simulink model "W01_Base_Map_cs"  (R2019a)
settings: Solver=FixedStepDiscrete  StartTime=0.0  StopTime=40  FixedStep=1/20  RelTol=1e-3
PreLoadFcn:
  | mbxruntime.callbacks.PreLoadFcn(bdroot);
  | check_NUTS_defined
  | model_closed = 0;
  | assignin('base',['model_closed_' bdroot],false);
PostLoadFcn:
  | mbxruntime.callbacks.PostLoadFcn(bdroot);
InitFcn:
  | mbxruntime.callbacks.InitFcn(bdroot);
StartFcn:
  | mbxruntime.callbacks.StartFcn(bdroot);
StopFcn:
  | mbxruntime.callbacks.StopFcn(bdroot);;
  | 
model workspace: external: MAT-File .\W01_Base_Map_cs_hws.mat (data not in the file)
undefined symbols (not defined in the file or in its folder): DiscIntNeverNeededParam, InitImageOutputDir, mbxruntime, tabledata, W01_Base_Map_cs_328ec7e3a8cd5b54, W01_Base_Map_cs_423c72fa17799c7f, W01_Base_Map_cs_514c2dea2cdbe680, W01_Base_Map_cs_51d6e6e467bedba1, W01_Base_Map_cs_563ebd29d1fd6c09, W01_Base_Map_cs_57ea59d0358dab77, W01_Base_Map_cs_669d1acb174df2b9, W01_Base_Map_cs_774a522413284ef7, W01_Base_Map_cs_9538d35a279fbe4e, W01_Base_Map_cs_9f504bb84aebc2fd, W01_Base_Map_cs_a242ed7539861165, W01_Base_Map_cs_ae41b72d7e14f81d, W01_Base_Map_cs_Audi_A8_Sedan_1_Path_pathUniqueID, W01_Base_Map_cs_b5931a786e299506, W01_Base_Map_cs_b7f45a070fa6e639, W01_Base_Map_cs_c02beb48492dde12, W01_Base_Map_cs_c75b75e9f6b035bf, W01_Base_Map_cs_cf83ac8e8b053cbf, W01_Base_Map_cs_Child_RegularAni_1_Path_pathUniqueID, W01_Base_Map_cs_Child_RegularAni_2_Path_pathUniqueID, W01_Base_Map_cs_Citroen_C3_Hatchback_1_Path_pathUniqueID, W01_Base_Map_cs_d4423fcf1c0d6fc4, W01_Base_Map_cs_df133aa86d9852fe, W01_Base_Map_cs_Female_RegularAni_1_Path_pathUniqueID, W01_Base_Map_cs_Male_RegularAni_1_Path_pathUniqueID, W01_Base_Map_cs_Male_RegularAni_2_Path_pathUniqueID
libraries: simulink_extras x41, adeye_lib x15, simulink x10, dspindex x6, PreScanSimulinkLibrary x4, sharedtransform x3, robotcorelib x1, PreScanUsefulBlocks x1
(part 9 of 11)

== system W01_Base_Map_cs/Ford_Fiesta_Hatchback_1/AIR_1_Demux ==
  AIR : Inport
  Activate_Switch : Subsystem
      mask Display: text(5,10,'')
  Bus Selector : BusSelector  OutputSignals=DATA.Range,DATA.Azimuth,DATA.Elevation,DATA.ID,DATA.Velocity,DATA.Heading
  Data Type Conversion : DataTypeConversion  OutDataTypeStr=double
  For Iterator : ForIterator  ResetStates=reset  IterationLimit=detectableObjects
  Selector : Selector  InputPortWidth=detectableObjects  IndexOptions=Index vector (port)  Indices=[1 3]  OutputSizes=1
  Signal2ArrayOfSignals1 : Subsystem  mask{VECTORLENGTH=detectableObjects}
      mask prompts: VECTORLENGTH "Length of vector"
  Signal2ArrayOfSignals2 : Subsystem  mask{VECTORLENGTH=detectableObjects}
      mask prompts: VECTORLENGTH "Length of vector"
  Signal2ArrayOfSignals3 : Subsystem  mask{VECTORLENGTH=detectableObjects}
      mask prompts: VECTORLENGTH "Length of vector"
  Signal2ArrayOfSignals4 : Subsystem  mask{VECTORLENGTH=detectableObjects}
      mask prompts: VECTORLENGTH "Length of vector"
  Signal2ArrayOfSignals5 : Subsystem  mask{VECTORLENGTH=detectableObjects}
      mask prompts: VECTORLENGTH "Length of vector"
  Signal2ArrayOfSignals6 : Subsystem  mask{VECTORLENGTH=detectableObjects}
      mask prompts: VECTORLENGTH "Length of vector"
  Range [m] : Outport
  Azimuth [deg] : Outport  Port=2
  Elevation [deg] : Outport  Port=3
  ID [-] : Outport  Port=4
  Velocity [m/s] : Outport  Port=5
  Heading [deg] : Outport  Port=6
  wires:
  Data Type Conversion/1 -> ID [-]/1
  Bus Selector/6 -> Signal2ArrayOfSignals6/2(Element)  "<Heading>"
  Signal2ArrayOfSignals6/1(ArrayofElements) -> Activate_Switch/2(Heading)
  Bus Selector/5 -> Signal2ArrayOfSignals5/2(Element)  "<Velocity>"
  Signal2ArrayOfSignals5/1(ArrayofElements) -> Velocity [m/s]/1
  Bus Selector/4 -> Signal2ArrayOfSignals4/2(Element)  "<ID>"
  Signal2ArrayOfSignals4/1(ArrayofElements) -> Data Type Conversion/1, Activate_Switch/1(BeamID)
  Bus Selector/3 -> Signal2ArrayOfSignals3/2(Element)  "<Elevation>"
  Signal2ArrayOfSignals3/1(ArrayofElements) -> Elevation [deg]/1
  Bus Selector/2 -> Signal2ArrayOfSignals1/2(Element)  "<Azimuth>"
  Signal2ArrayOfSignals1/1(ArrayofElements) -> Azimuth [deg]/1
  Signal2ArrayOfSignals2/1(ArrayofElements) -> Range [m]/1
  Bus Selector/1 -> Signal2ArrayOfSignals2/2(Element)  "<Range>"
  Selector/1 -> Bus Selector/1
  For Iterator/1 -> Signal2ArrayOfSignals6/1(LoopIndex), Signal2ArrayOfSignals5/1(LoopIndex), Signal2ArrayOfSignals4/1(LoopIndex), Signal2ArrayOfSignals3/1(LoopIndex), Signal2ArrayOfSignals1/1(LoopIndex), Signal2ArrayOfSignals2/1(LoopIndex), Selector/2
  AIR/1 -> Selector/1
  Activate_Switch/1(On/Off) -> Heading [deg]/1

== system W01_Base_Map_cs/Ford_Fiesta_Hatchback_1/Car_Pos_and_Orient ==
  In1 : Inport
  In2 : Inport  Port=2
  In3 : Inport  Port=3
  In4 : Inport  Port=4
  In5 : Inport  Port=5
  In6 : Inport  Port=6
  Data Type Conversion : DataTypeConversion
  Data Type Conversion1 : DataTypeConversion
  Data Type Conversion2 : DataTypeConversion
  Degrees to Radians1 : simulink_extras/Transformations/Degrees to Radians
  Degrees to Radians2 : simulink_extras/Transformations/Degrees to Radians
  Degrees to Radians5 : simulink_extras/Transformations/Degrees to Radians
  Mux : Mux
  Rotation Angles to Quaternions : sharedtransform/Rotation Angles to Quaternions  rotationOrder=XYZ  aMode=aMode
      settings: SourceProductName=Aerospace Blockset  SourceProductBaseCode=AE
  Vector Concatenate2 : Concatenate  NumInputs=3
  Out1 : Outport
  wires:
  Degrees to Radians1/1 -> Vector Concatenate2/2
  Degrees to Radians5/1 -> Vector Concatenate2/1
  Vector Concatenate2/1 -> Rotation Angles to Quaternions/1
  Degrees to Radians2/1 -> Vector Concatenate2/3
  In1/1 -> Data Type Conversion/1
  In2/1 -> Data Type Conversion1/1
  In3/1 -> Data Type Conversion2/1
  In4/1 -> Degrees to Radians5/1
  In5/1 -> Degrees to Radians1/1
  In6/1 -> Degrees to Radians2/1
  Data Type Conversion/1 -> Mux/1
  Data Type Conversion1/1 -> Mux/2
  Data Type Conversion2/1 -> Mux/3
  Rotation Angles to Quaternions/1 -> Mux/4
  Mux/1 -> Out1/1

== system W01_Base_Map_cs/Ford_Fiesta_Hatchback_1/Dynamics_Empty ==
  note: For state mode 'Dynamic' positions
      | are not taken into account, as they
      | are computed by integrating velocity.
      | Click annotation for Help.
  Ground_{1..9} (9 alike) : Ground
  MuxState : Subsystem  Tag=mux/State  mask(Empty Dynamics State Block){positioningmode=on, TimeStep=1/20}
      mask prompts: positioningmode "Positioning Mode"; TimeStep "Auto Assigned: Time Step [s]"
      mask help:
      | Build the state of an actor based on user input.
      | The user can either use positioning mode or dynamics mode.
      | - When using positioning mode the position and orientation of the actor are set directly based on the input. Expected input is relative to the initial position and orientation of the actor. It's also possible to specify the velocity of the actor, though this input isn't used, only passed on.
      | - When using dynamics mode the position input is ignored. Expected input is velocity and orientation. The velocity is relative the current orientation of the actor, while orientation is relative to its initial orientation. The position of the actor is calculated based on the velocity and orientation given.
      settings: DeleteFcn=PreScanBlockDeleteFcn;
  STATE_Ford_Fiesta_Hatchback_1 : Subsystem  Tag=mux/StatePort  Priority=0  LoadFcn=load PrescanStateActuatorData  mask(PreScan Sink Block: State){x0=W01_Base_Map_cs_df133aa86d9852fe, y0=W01_Base_Map_cs_ae41b72d7e14f81d, z0=W01_Base_Map_cs_669d1acb174df2b9, Roll0=W01_Base_Map_cs_423c72fa17799c7f, Pitch0=W01_Base_Map_cs_c75b75e9f6b035bf, Yaw0=W01_Base_Map_cs_774a522413284ef7, TimeStep=1/20}
      mask prompts: x0 "Ini x-position VEHICLE wrt GLOBAL axis system [m]"; y0 "Ini y-position VEHICLE wrt GLOBAL axis system [m]"; z0 "Ini z-position VEHICLE wrt GLOBAL axis system [m]"; Roll0 "Ini roll-angle BODY wrt VEHICLE axis system [deg]"; Pitch0 "Ini pitch-angle BODY wrt VEHICLE axis system [deg]"; Yaw0 "Ini yaw-angle VEHICLE wrt GLOBAL axis system [deg]"; TimeStep "Auto-Assigned: Upload Period [s]"
      mask help:
      | The Actor State contains a vector signal of size (9x1), containing the following signals:
      |
      | -  Position                  (x,y,z)                                     [m]
      | -  Velocity                  (vx,vy,vz)                               [m/s]
      | -  Angles                    (Roll, Pitch, Yaw)                   [rad]
      |
      | The Actor state is defined in the global axis system.
      | The state is superponed on the Initial position defined in the GUI.
      |
      | For more information, please click Help.
      settings: DeleteFcn=PreScanBlockDeleteFcn;
      mask Help: eval('openHelp(222)')
      mask Display: image(imread('State.png'))
  State : Outport  Tag=outport/StateOutport  SampleTime=1/20
  wires:
  Ground_9/1 -> MuxState/4(dx [m/s])
  MuxState/1(state) -> STATE_Ford_Fiesta_Hatchback_1/1(State)
  STATE_Ford_Fiesta_Hatchback_1/1(StateBus) -> State/1
  Ground_1/1 -> MuxState/1(x [m])
  Ground_2/1 -> MuxState/2(y [m])
  Ground_3/1 -> MuxState/3(z [m])
  Ground_4/1 -> MuxState/5(dy [m/s])
  Ground_5/1 -> MuxState/6(dz [m/s])
  Ground_6/1 -> MuxState/7(R [rad])
  Ground_7/1 -> MuxState/8(P [rad])
  Ground_8/1 -> MuxState/9(Y [rad])

== system W01_Base_Map_cs/Ford_Fiesta_Hatchback_1/SELF_Demux ==
  SELF : Inport  OutDataTypeStr=Bus: PRESCAN_SELFSENSORDATA
  Bus Selector : BusSelector  OutputSignals=PositionX,PositionY,PositionZ,OrientationRoll,OrientationPitch,OrientationYaw,Velocity,Yaw_rate,Lat,Long,Alt
  Demux2 : Demux  Outputs=3
  Gain : Gain  Gain=180/pi
  Gain1 : Gain  Gain=180/pi
  Vector Concatenate1 : Concatenate  NumInputs=3
  compas converter : Subsystem
  x [m] : Outport
  y [m] : Outport  Port=2
  z [m] : Outport  Port=3
  rotx [deg] : Outport  Port=4
  roty [deg] : Outport  Port=5
  rotz [deg] : Outport  Port=6
  GPS lat [deg] : Outport  Port=7
  GPS long [deg] : Outport  Port=8
  GPS alt [m] : Outport  Port=9
  velocity [m/s] : Outport  Port=10
  heading [deg] : Outport  Port=11
  yaw rate [deg/s] : Outport  Port=12
  wires:
  Bus Selector/11 -> GPS alt [m]/1  "<Alt>"
  Bus Selector/10 -> GPS long [deg]/1  "<Long>"
  Bus Selector/9 -> GPS lat [deg]/1  "<Lat>"
  Bus Selector/8 -> Gain1/1  "<Yaw_rate>"
  Bus Selector/7 -> velocity [m/s]/1  "<Velocity>"
  Bus Selector/6 -> compas converter/1(rotz [rad]), Vector Concatenate1/3  "<OrientationYaw>"
  Bus Selector/5 -> Vector Concatenate1/2  "<OrientationPitch>"
  Bus Selector/4 -> Vector Concatenate1/1  "<OrientationRoll>"
  Vector Concatenate1/1 -> Gain/1
  Bus Selector/3 -> z [m]/1  "<PositionZ>"
  Bus Selector/2 -> y [m]/1  "<PositionY>"
  Bus Selector/1 -> x [m]/1  "<PositionX>"
  SELF/1 -> Bus Selector/1
  Gain/1 -> Demux2/1
  Demux2/1 -> rotx [deg]/1
  Demux2/2 -> roty [deg]/1
  Demux2/3 -> rotz [deg]/1
  compas converter/1(heading [deg]) -> heading [deg]/1
  Gain1/1 -> yaw rate [deg/s]/1

== system W01_Base_Map_cs/Male_RegularAni_1/Animation ==
  In1 : Inport
  Bus Creator : BusCreator  Inputs=2  OutDataTypeStr=Bus: PRESCAN_ANIMACTUATORDATA  NonVirtualBus=on
  Bus Selector : BusSelector  OutputSignals=VelocityX,VelocityY,VelocityZ
  Data Type Conversion : DataTypeConversion  OutDataTypeStr=int32
  Mux : Mux  Inputs=3
  Product : Product  RndMeth=Zero
  RunningScale : Constant  Value=RunningScale
  Switch : Switch  Threshold=2
  WalkingScale : Constant  Value=WalkingScale
  animation mode : Subsystem
  elapsed track : Subsystem
  Out1 : Outport
  wires:
  Switch/1 -> Product/1
  WalkingScale/1 -> Switch/3
  RunningScale/1 -> Switch/1
  elapsed track/1(s) -> Product/2  "Time"
  Product/1 -> Bus Creator/2  "Time"
  Mux/1 -> elapsed track/1(vel), animation mode/1(vel)
  Bus Selector/1 -> Mux/1  "<VelocityX>"
  Bus Selector/2 -> Mux/2  "<VelocityY>"
  Bus Selector/3 -> Mux/3  "<VelocityZ>"
  animation mode/1(mode) -> Switch/2, Data Type Conversion/1
  In1/1 -> Bus Selector/1
  Bus Creator/1 -> Out1/1
  Data Type Conversion/1 -> Bus Creator/1  "Index"

== system W01_Base_Map_cs/Male_RegularAni_1/SELF_Demux ==
  SELF : Inport  OutDataTypeStr=Bus: PRESCAN_SELFSENSORDATA
  Bus Selector : BusSelector  OutputSignals=PositionX,PositionY,PositionZ,OrientationRoll,OrientationPitch,OrientationYaw,Velocity,Yaw_rate,Lat,Long,Alt
  Demux2 : Demux  Outputs=3
  Gain : Gain  Gain=180/pi
  Gain1 : Gain  Gain=180/pi
  Vector Concatenate1 : Concatenate  NumInputs=3
  compas converter : Subsystem
  x [m] : Outport
  y [m] : Outport  Port=2
  z [m] : Outport  Port=3
  rotx [deg] : Outport  Port=4
  roty [deg] : Outport  Port=5
  rotz [deg] : Outport  Port=6
  GPS lat [deg] : Outport  Port=7
  GPS long [deg] : Outport  Port=8
  GPS alt [m] : Outport  Port=9
  velocity [m/s] : Outport  Port=10
  heading [deg] : Outport  Port=11
  yaw rate [deg/s] : Outport  Port=12
  wires:
  Bus Selector/11 -> GPS alt [m]/1  "<Alt>"
  Bus Selector/10 -> GPS long [deg]/1  "<Long>"
  Bus Selector/9 -> GPS lat [deg]/1  "<Lat>"
  Bus Selector/8 -> Gain1/1  "<Yaw_rate>"
  Bus Selector/7 -> velocity [m/s]/1  "<Velocity>"
  Bus Selector/6 -> compas converter/1(rotz [rad]), Vector Concatenate1/3  "<OrientationYaw>"
  Bus Selector/5 -> Vector Concatenate1/2  "<OrientationPitch>"
  Bus Selector/4 -> Vector Concatenate1/1  "<OrientationRoll>"
  Vector Concatenate1/1 -> Gain/1
  Bus Selector/3 -> z [m]/1  "<PositionZ>"
  Bus Selector/2 -> y [m]/1  "<PositionY>"
  Bus Selector/1 -> x [m]/1  "<PositionX>"
  SELF/1 -> Bus Selector/1
  Gain/1 -> Demux2/1
  Demux2/1 -> rotx [deg]/1
  Demux2/2 -> roty [deg]/1
  Demux2/3 -> rotz [deg]/1
  compas converter/1(heading [deg]) -> heading [deg]/1
  Gain1/1 -> yaw rate [deg/s]/1

== system W01_Base_Map_cs/Male_RegularAni_1/VISUColorRegion_Lower_Body_Mux ==
  RGB [-,-,-] : Inport
  Bus Creator : BusCreator  Inputs=4  OutDataTypeStr=Bus: PRESCAN_COLOR_DATA  NonVirtualBus=on
  Constant : Constant  Value=255  OutDataTypeStr=uint8
  Data Type Conversion : DataTypeConversion  OutDataTypeStr=uint8
  Data Type Conversion1 : DataTypeConversion  OutDataTypeStr=uint8
  Data Type Conversion2 : DataTypeConversion  OutDataTypeStr=uint8
  Demux : Demux  Outputs=3
  ColorRegion : Outport  OutDataTypeStr=Bus: PRESCAN_COLOR_DATA  PortDimensions=1
  wires:
  Constant/1 -> Bus Creator/4  "A"
  Data Type Conversion2/1 -> Bus Creator/3  "B"
  Data Type Conversion1/1 -> Bus Creator/2  "G"
  Data Type Conversion/1 -> Bus Creator/1  "R"
  Demux/3 -> Data Type Conversion2/1  "B"
  Demux/2 -> Data Type Conversion1/1  "G"
  Demux/1 -> Data Type Conversion/1  "R"
  RGB [-,-,-]/1 -> Demux/1
  Bus Creator/1 -> ColorRegion/1

== system W01_Base_Map_cs/Male_RegularAni_1/VISUColorRegion_Shoes_Mux ==
  RGB [-,-,-] : Inport
  Bus Creator : BusCreator  Inputs=4  OutDataTypeStr=Bus: PRESCAN_COLOR_DATA  NonVirtualBus=on
  Constant : Constant  Value=255  OutDataTypeStr=uint8
  Data Type Conversion : DataTypeConversion  OutDataTypeStr=uint8
  Data Type Conversion1 : DataTypeConversion  OutDataTypeStr=uint8
  Data Type Conversion2 : DataTypeConversion  OutDataTypeStr=uint8
  Demux : Demux  Outputs=3
  ColorRegion : Outport  OutDataTypeStr=Bus: PRESCAN_COLOR_DATA  PortDimensions=1
  wires:
  Constant/1 -> Bus Creator/4  "A"
  Data Type Conversion2/1 -> Bus Creator/3  "B"
  Data Type Conversion1/1 -> Bus Creator/2  "G"
  Data Type Conversion/1 -> Bus Creator/1  "R"
  Demux/3 -> Data Type Conversion2/1  "B"
  Demux/2 -> Data Type Conversion1/1  "G"
  Demux/1 -> Data Type Conversion/1  "R"
  RGB [-,-,-]/1 -> Demux/1
  Bus Creator/1 -> ColorRegion/1

== system W01_Base_Map_cs/Male_RegularAni_1/VISUColorRegion_Upper_Body_Mux ==
  RGB [-,-,-] : Inport
  Bus Creator : BusCreator  Inputs=4  OutDataTypeStr=Bus: PRESCAN_COLOR_DATA  NonVirtualBus=on
  Constant : Constant  Value=255  OutDataTypeStr=uint8
  Data Type Conversion : DataTypeConversion  OutDataTypeStr=uint8
  Data Type Conversion1 : DataTypeConversion  OutDataTypeStr=uint8
  Data Type Conversion2 : DataTypeConversion  OutDataTypeStr=uint8
  Demux : Demux  Outputs=3
  ColorRegion : Outport  OutDataTypeStr=Bus: PRESCAN_COLOR_DATA  PortDimensions=1
  wires:
  Constant/1 -> Bus Creator/4  "A"
  Data Type Conversion2/1 -> Bus Creator/3  "B"
  Data Type Conversion1/1 -> Bus Creator/2  "G"
  Data Type Conversion/1 -> Bus Creator/1  "R"
  Demux/3 -> Data Type Conversion2/1  "B"
  Demux/2 -> Data Type Conversion1/1  "G"
  Demux/1 -> Data Type Conversion/1  "R"
  RGB [-,-,-]/1 -> Demux/1
  Bus Creator/1 -> ColorRegion/1

== system W01_Base_Map_cs/Male_RegularAni_2/Animation ==
  In1 : Inport
  Bus Creator : BusCreator  Inputs=2  OutDataTypeStr=Bus: PRESCAN_ANIMACTUATORDATA  NonVirtualBus=on
  Bus Selector : BusSelector  OutputSignals=VelocityX,VelocityY,VelocityZ
  Data Type Conversion : DataTypeConversion  OutDataTypeStr=int32
  Mux : Mux  Inputs=3
  Product : Product  RndMeth=Zero
  RunningScale : Constant  Value=RunningScale
  Switch : Switch  Threshold=2
  WalkingScale : Constant  Value=WalkingScale
  animation mode : Subsystem
  elapsed track : Subsystem
  Out1 : Outport
  wires:
  Switch/1 -> Product/1
  WalkingScale/1 -> Switch/3
  RunningScale/1 -> Switch/1
  elapsed track/1(s) -> Product/2  "Time"
  Product/1 -> Bus Creator/2  "Time"
  Mux/1 -> elapsed track/1(vel), animation mode/1(vel)
  Bus Selector/1 -> Mux/1  "<VelocityX>"
  Bus Selector/2 -> Mux/2  "<VelocityY>"
  Bus Selector/3 -> Mux/3  "<VelocityZ>"
  animation mode/1(mode) -> Switch/2, Data Type Conversion/1
  In1/1 -> Bus Selector/1
  Bus Creator/1 -> Out1/1
  Data Type Conversion/1 -> Bus Creator/1  "Index"

== system W01_Base_Map_cs/Male_RegularAni_2/SELF_Demux ==
  SELF : Inport  OutDataTypeStr=Bus: PRESCAN_SELFSENSORDATA
  Bus Selector : BusSelector  OutputSignals=PositionX,PositionY,PositionZ,OrientationRoll,OrientationPitch,OrientationYaw,Velocity,Yaw_rate,Lat,Long,Alt
  Demux2 : Demux  Outputs=3
  Gain : Gain  Gain=180/pi
  Gain1 : Gain  Gain=180/pi
  Vector Concatenate1 : Concatenate  NumInputs=3
  compas converter : Subsystem
  x [m] : Outport
  y [m] : Outport  Port=2
  z [m] : Outport  Port=3
  rotx [deg] : Outport  Port=4
  roty [deg] : Outport  Port=5
  rotz [deg] : Outport  Port=6
  GPS lat [deg] : Outport  Port=7
  GPS long [deg] : Outport  Port=8
  GPS alt [m] : Outport  Port=9
  velocity [m/s] : Outport  Port=10
  heading [deg] : Outport  Port=11
  yaw rate [deg/s] : Outport  Port=12
  wires:
  Bus Selector/11 -> GPS alt [m]/1  "<Alt>"
  Bus Selector/10 -> GPS long [deg]/1  "<Long>"
  Bus Selector/9 -> GPS lat [deg]/1  "<Lat>"
  Bus Selector/8 -> Gain1/1  "<Yaw_rate>"
  Bus Selector/7 -> velocity [m/s]/1  "<Velocity>"
  Bus Selector/6 -> compas converter/1(rotz [rad]), Vector Concatenate1/3  "<OrientationYaw>"
  Bus Selector/5 -> Vector Concatenate1/2  "<OrientationPitch>"
  Bus Selector/4 -> Vector Concatenate1/1  "<OrientationRoll>"
  Vector Concatenate1/1 -> Gain/1
  Bus Selector/3 -> z [m]/1  "<PositionZ>"
  Bus Selector/2 -> y [m]/1  "<PositionY>"
  Bus Selector/1 -> x [m]/1  "<PositionX>"
  SELF/1 -> Bus Selector/1
  Gain/1 -> Demux2/1
  Demux2/1 -> rotx [deg]/1
  Demux2/2 -> roty [deg]/1
  Demux2/3 -> rotz [deg]/1
  compas converter/1(heading [deg]) -> heading [deg]/1
  Gain1/1 -> yaw rate [deg/s]/1

== system W01_Base_Map_cs/Male_RegularAni_2/VISUColorRegion_Lower_Body_Mux ==
  RGB [-,-,-] : Inport
  Bus Creator : BusCreator  Inputs=4  OutDataTypeStr=Bus: PRESCAN_COLOR_DATA  NonVirtualBus=on
  Constant : Constant  Value=255  OutDataTypeStr=uint8
  Data Type Conversion : DataTypeConversion  OutDataTypeStr=uint8
  Data Type Conversion1 : DataTypeConversion  OutDataTypeStr=uint8
  Data Type Conversion2 : DataTypeConversion  OutDataTypeStr=uint8
  Demux : Demux  Outputs=3
  ColorRegion : Outport  OutDataTypeStr=Bus: PRESCAN_COLOR_DATA  PortDimensions=1
  wires:
  Constant/1 -> Bus Creator/4  "A"
  Data Type Conversion2/1 -> Bus Creator/3  "B"
  Data Type Conversion1/1 -> Bus Creator/2  "G"
  Data Type Conversion/1 -> Bus Creator/1  "R"
  Demux/3 -> Data Type Conversion2/1  "B"
  Demux/2 -> Data Type Conversion1/1  "G"
  Demux/1 -> Data Type Conversion/1  "R"
  RGB [-,-,-]/1 -> Demux/1
  Bus Creator/1 -> ColorRegion/1

== system W01_Base_Map_cs/Male_RegularAni_2/VISUColorRegion_Shoes_Mux ==
  RGB [-,-,-] : Inport
  Bus Creator : BusCreator  Inputs=4  OutDataTypeStr=Bus: PRESCAN_COLOR_DATA  NonVirtualBus=on
  Constant : Constant  Value=255  OutDataTypeStr=uint8
  Data Type Conversion : DataTypeConversion  OutDataTypeStr=uint8
  Data Type Conversion1 : DataTypeConversion  OutDataTypeStr=uint8
  Data Type Conversion2 : DataTypeConversion  OutDataTypeStr=uint8
  Demux : Demux  Outputs=3
  ColorRegion : Outport  OutDataTypeStr=Bus: PRESCAN_COLOR_DATA  PortDimensions=1
  wires:
  Constant/1 -> Bus Creator/4  "A"
  Data Type Conversion2/1 -> Bus Creator/3  "B"
  Data Type Conversion1/1 -> Bus Creator/2  "G"
  Data Type Conversion/1 -> Bus Creator/1  "R"
  Demux/3 -> Data Type Conversion2/1  "B"
  Demux/2 -> Data Type Conversion1/1  "G"
  Demux/1 -> Data Type Conversion/1  "R"
  RGB [-,-,-]/1 -> Demux/1
  Bus Creator/1 -> ColorRegion/1

== system W01_Base_Map_cs/Male_RegularAni_2/VISUColorRegion_Upper_Body_Mux ==
  RGB [-,-,-] : Inport
  Bus Creator : BusCreator  Inputs=4  OutDataTypeStr=Bus: PRESCAN_COLOR_DATA  NonVirtualBus=on
  Constant : Constant  Value=255  OutDataTypeStr=uint8
  Data Type Conversion : DataTypeConversion  OutDataTypeStr=uint8
  Data Type Conversion1 : DataTypeConversion  OutDataTypeStr=uint8
  Data Type Conversion2 : DataTypeConversion  OutDataTypeStr=uint8
  Demux : Demux  Outputs=3
  ColorRegion : Outport  OutDataTypeStr=Bus: PRESCAN_COLOR_DATA  PortDimensions=1
  wires:
  Constant/1 -> Bus Creator/4  "A"
  Data Type Conversion2/1 -> Bus Creator/3  "B"
  Data Type Conversion1/1 -> Bus Creator/2  "G"
  Data Type Conversion/1 -> Bus Creator/1  "R"
  Demux/3 -> Data Type Conversion2/1  "B"
  Demux/2 -> Data Type Conversion1/1  "G"
  Demux/1 -> Data Type Conversion/1  "R"
  RGB [-,-,-]/1 -> Demux/1
  Bus Creator/1 -> ColorRegion/1

== system W01_Base_Map_cs/TrafficLightRoadSideNL_1/Green_Mux ==
  MSCD [Cd] : Inport
  Position (xyz) [m] : Inport  Port=2
  Orientation (RPY) [deg] : Inport  Port=3
  Color [-] : Inport  Port=4
  TextureResourceID [-] : Inport  Port=5
  Bus Creator : BusCreator  Inputs='Intensity','Position','Orientation','Color','TextureResourceID'  OutDataTypeStr=Bus: PRESCAN_VISULIGHTACTUATOR_DATA  NonVirtualBus=on
  Bus Creator1 : BusCreator  Inputs=3  OutDataTypeStr=Bus: PRESCAN_RGB_DATA  NonVirtualBus=on
  Bus Creator2 : BusCreator  Inputs=3  OutDataTypeStr=Bus: PRESCAN_RPY_DATA  NonVirtualBus=on
  Bus Creator3 : BusCreator  Inputs=3  OutDataTypeStr=Bus: PRESCAN_XYZ_DATA  NonVirtualBus=on
  Data Type Conversion : DataTypeConversion  OutDataTypeStr=int32  RndMeth=Nearest
  Degrees to Radians : simulink_extras/Transformations/Degrees to Radians
  Demux : Demux  Outputs=3
  Demux1 : Demux  Outputs=3
  Demux2 : Demux  Outputs=3
  Lights : Outport
  wires:
  TextureResourceID [-]/1 -> Data Type Conversion/1  "TextureResourceID"
  MSCD [Cd]/1 -> Bus Creator/1  "Intensity"
  Bus Creator/1 -> Lights/1
  Demux/1 -> Bus Creator1/1  "R"
  Demux/2 -> Bus Creator1/2  "G"
  Demux/3 -> Bus Creator1/3  "B"
  Color [-]/1 -> Demux/1  "Color"
  Bus Creator1/1 -> Bus Creator/4  "Color"
  Demux1/1 -> Bus Creator2/1  "Roll"
  Demux1/2 -> Bus Creator2/2  "Pitch"
  Demux1/3 -> Bus Creator2/3  "Yaw"
  Orientation (RPY) [deg]/1 -> Degrees to Radians/1  "Orientation"
  Bus Creator2/1 -> Bus Creator/3  "Orientation"
  Demux2/1 -> Bus Creator3/1  "X"
  Demux2/2 -> Bus Creator3/2  "Y"
  Demux2/3 -> Bus Creator3/3  "Z"
  Position (xyz) [m]/1 -> Demux2/1  "Position"
  Bus Creator3/1 -> Bus Creator/2  "Position"
  Data Type Conversion/1 -> Bus Creator/5  "TextureResourceID"
  Degrees to Radians/1 -> Demux1/1

== system W01_Base_Map_cs/TrafficLightRoadSideNL_1/Orange_Mux ==
  MSCD [Cd] : Inport
  Position (xyz) [m] : Inport  Port=2
  Orientation (RPY) [deg] : Inport  Port=3
  Color [-] : Inport  Port=4
  TextureResourceID [-] : Inport  Port=5
  Bus Creator : BusCreator  Inputs='Intensity','Position','Orientation','Color','TextureResourceID'  OutDataTypeStr=Bus: PRESCAN_VISULIGHTACTUATOR_DATA  NonVirtualBus=on
  Bus Creator1 : BusCreator  Inputs=3  OutDataTypeStr=Bus: PRESCAN_RGB_DATA  NonVirtualBus=on
  Bus Creator2 : BusCreator  Inputs=3  OutDataTypeStr=Bus: PRESCAN_RPY_DATA  NonVirtualBus=on
  Bus Creator3 : BusCreator  Inputs=3  OutDataTypeStr=Bus: PRESCAN_XYZ_DATA  NonVirtualBus=on
  Data Type Conversion : DataTypeConversion  OutDataTypeStr=int32  RndMeth=Nearest
  Degrees to Radians : simulink_extras/Transformations/Degrees to Radians
  Demux : Demux  Outputs=3
  Demux1 : Demux  Outputs=3
  Demux2 : Demux  Outputs=3
  Lights : Outport
  wires:
  TextureResourceID [-]/1 -> Data Type Conversion/1  "TextureResourceID"
  MSCD [Cd]/1 -> Bus Creator/1  "Intensity"
  Bus Creator/1 -> Lights/1
  Demux/1 -> Bus Creator1/1  "R"
  Demux/2 -> Bus Creator1/2  "G"
  Demux/3 -> Bus Creator1/3  "B"
  Color [-]/1 -> Demux/1  "Color"
  Bus Creator1/1 -> Bus Creator/4  "Color"
  Demux1/1 -> Bus Creator2/1  "Roll"
  Demux1/2 -> Bus Creator2/2  "Pitch"
  Demux1/3 -> Bus Creator2/3  "Yaw"
  Orientation (RPY) [deg]/1 -> Degrees to Radians/1  "Orientation"
  Bus Creator2/1 -> Bus Creator/3  "Orientation"
  Demux2/1 -> Bus Creator3/1  "X"
  Demux2/2 -> Bus Creator3/2  "Y"
  Demux2/3 -> Bus Creator3/3  "Z"
  Position (xyz) [m]/1 -> Demux2/1  "Position"
  Bus Creator3/1 -> Bus Creator/2  "Position"
  Data Type Conversion/1 -> Bus Creator/5  "TextureResourceID"
  Degrees to Radians/1 -> Demux1/1

== system W01_Base_Map_cs/TrafficLightRoadSideNL_1/Red_Mux ==
  MSCD [Cd] : Inport
  Position (xyz) [m] : Inport  Port=2
  Orientation (RPY) [deg] : Inport  Port=3
  Color [-] : Inport  Port=4
  TextureResourceID [-] : Inport  Port=5
  Bus Creator : BusCreator  Inputs='Intensity','Position','Orientation','Color','TextureResourceID'  OutDataTypeStr=Bus: PRESCAN_VISULIGHTACTUATOR_DATA  NonVirtualBus=on
  Bus Creator1 : BusCreator  Inputs=3  OutDataTypeStr=Bus: PRESCAN_RGB_DATA  NonVirtualBus=on
  Bus Creator2 : BusCreator  Inputs=3  OutDataTypeStr=Bus: PRESCAN_RPY_DATA  NonVirtualBus=on
  Bus Creator3 : BusCreator  Inputs=3  OutDataTypeStr=Bus: PRESCAN_XYZ_DATA  NonVirtualBus=on
  Data Type Conversion : DataTypeConversion  OutDataTypeStr=int32  RndMeth=Nearest
  Degrees to Radians : simulink_extras/Transformations/Degrees to Radians
  Demux : Demux  Outputs=3
  Demux1 : Demux  Outputs=3
  Demux2 : Demux  Outputs=3
  Lights : Outport
  wires:
  TextureResourceID [-]/1 -> Data Type Conversion/1  "TextureResourceID"
  MSCD [Cd]/1 -> Bus Creator/1  "Intensity"
  Bus Creator/1 -> Lights/1
  Demux/1 -> Bus Creator1/1  "R"
  Demux/2 -> Bus Creator1/2  "G"
  Demux/3 -> Bus Creator1/3  "B"
  Color [-]/1 -> Demux/1  "Color"
  Bus Creator1/1 -> Bus Creator/4  "Color"
  Demux1/1 -> Bus Creator2/1  "Roll"
  Demux1/2 -> Bus Creator2/2  "Pitch"
  Demux1/3 -> Bus Creator2/3  "Yaw"
  Orientation (RPY) [deg]/1 -> Degrees to Radians/1  "Orientation"
  Bus Creator2/1 -> Bus Creator/3  "Orientation"
  Demux2/1 -> Bus Creator3/1  "X"
  Demux2/2 -> Bus Creator3/2  "Y"
  Demux2/3 -> Bus Creator3/3  "Z"
  Position (xyz) [m]/1 -> Demux2/1  "Position"
  Bus Creator3/1 -> Bus Creator/2  "Position"
  Data Type Conversion/1 -> Bus Creator/5  "TextureResourceID"
  Degrees to Radians/1 -> Demux1/1

== system W01_Base_Map_cs/TrafficLightRoadSideNL_2/Green_Mux ==
  MSCD [Cd] : Inport
  Position (xyz) [m] : Inport  Port=2
  Orientation (RPY) [deg] : Inport  Port=3
  Color [-] : Inport  Port=4
  TextureResourceID [-] : Inport  Port=5
  Bus Creator : BusCreator  Inputs='Intensity','Position','Orientation','Color','TextureResourceID'  OutDataTypeStr=Bus: PRESCAN_VISULIGHTACTUATOR_DATA  NonVirtualBus=on
  Bus Creator1 : BusCreator  Inputs=3  OutDataTypeStr=Bus: PRESCAN_RGB_DATA  NonVirtualBus=on
  Bus Creator2 : BusCreator  Inputs=3  OutDataTypeStr=Bus: PRESCAN_RPY_DATA  NonVirtualBus=on
  Bus Creator3 : BusCreator  Inputs=3  OutDataTypeStr=Bus: PRESCAN_XYZ_DATA  NonVirtualBus=on
  Data Type Conversion : DataTypeConversion  OutDataTypeStr=int32  RndMeth=Nearest
  Degrees to Radians : simulink_extras/Transformations/Degrees to Radians
  Demux : Demux  Outputs=3
  Demux1 : Demux  Outputs=3
  Demux2 : Demux  Outputs=3
  Lights : Outport
  wires:
  TextureResourceID [-]/1 -> Data Type Conversion/1  "TextureResourceID"
  MSCD [Cd]/1 -> Bus Creator/1  "Intensity"
  Bus Creator/1 -> Lights/1
  Demux/1 -> Bus Creator1/1  "R"
  Demux/2 -> Bus Creator1/2  "G"
  Demux/3 -> Bus Creator1/3  "B"
  Color [-]/1 -> Demux/1  "Color"
  Bus Creator1/1 -> Bus Creator/4  "Color"
  Demux1/1 -> Bus Creator2/1  "Roll"
  Demux1/2 -> Bus Creator2/2  "Pitch"
  Demux1/3 -> Bus Creator2/3  "Yaw"
  Orientation (RPY) [deg]/1 -> Degrees to Radians/1  "Orientation"
  Bus Creator2/1 -> Bus Creator/3  "Orientation"
  Demux2/1 -> Bus Creator3/1  "X"
  Demux2/2 -> Bus Creator3/2  "Y"
  Demux2/3 -> Bus Creator3/3  "Z"
  Position (xyz) [m]/1 -> Demux2/1  "Position"
  Bus Creator3/1 -> Bus Creator/2  "Position"
  Data Type Conversion/1 -> Bus Creator/5  "TextureResourceID"
  Degrees to Radians/1 -> Demux1/1

== system W01_Base_Map_cs/TrafficLightRoadSideNL_2/Orange_Mux ==
  MSCD [Cd] : Inport
  Position (xyz) [m] : Inport  Port=2
  Orientation (RPY) [deg] : Inport  Port=3
  Color [-] : Inport  Port=4
  TextureResourceID [-] : Inport  Port=5
  Bus Creator : BusCreator  Inputs='Intensity','Position','Orientation','Color','TextureResourceID'  OutDataTypeStr=Bus: PRESCAN_VISULIGHTACTUATOR_DATA  NonVirtualBus=on
  Bus Creator1 : BusCreator  Inputs=3  OutDataTypeStr=Bus: PRESCAN_RGB_DATA  NonVirtualBus=on
  Bus Creator2 : BusCreator  Inputs=3  OutDataTypeStr=Bus: PRESCAN_RPY_DATA  NonVirtualBus=on
  Bus Creator3 : BusCreator  Inputs=3  OutDataTypeStr=Bus: PRESCAN_XYZ_DATA  NonVirtualBus=on
  Data Type Conversion : DataTypeConversion  OutDataTypeStr=int32  RndMeth=Nearest
  Degrees to Radians : simulink_extras/Transformations/Degrees to Radians
  Demux : Demux  Outputs=3
  Demux1 : Demux  Outputs=3
  Demux2 : Demux  Outputs=3
  Lights : Outport
  wires:
  TextureResourceID [-]/1 -> Data Type Conversion/1  "TextureResourceID"
  MSCD [Cd]/1 -> Bus Creator/1  "Intensity"
  Bus Creator/1 -> Lights/1
  Demux/1 -> Bus Creator1/1  "R"
  Demux/2 -> Bus Creator1/2  "G"
  Demux/3 -> Bus Creator1/3  "B"
  Color [-]/1 -> Demux/1  "Color"
  Bus Creator1/1 -> Bus Creator/4  "Color"
  Demux1/1 -> Bus Creator2/1  "Roll"
  Demux1/2 -> Bus Creator2/2  "Pitch"
  Demux1/3 -> Bus Creator2/3  "Yaw"
  Orientation (RPY) [deg]/1 -> Degrees to Radians/1  "Orientation"
  Bus Creator2/1 -> Bus Creator/3  "Orientation"
  Demux2/1 -> Bus Creator3/1  "X"
  Demux2/2 -> Bus Creator3/2  "Y"
  Demux2/3 -> Bus Creator3/3  "Z"
  Position (xyz) [m]/1 -> Demux2/1  "Position"
  Bus Creator3/1 -> Bus Creator/2  "Position"
  Data Type Conversion/1 -> Bus Creator/5  "TextureResourceID"
  Degrees to Radians/1 -> Demux1/1

== system W01_Base_Map_cs/TrafficLightRoadSideNL_2/Red_Mux ==
  MSCD [Cd] : Inport
  Position (xyz) [m] : Inport  Port=2
  Orientation (RPY) [deg] : Inport  Port=3
  Color [-] : Inport  Port=4
  TextureResourceID [-] : Inport  Port=5
  Bus Creator : BusCreator  Inputs='Intensity','Position','Orientation','Color','TextureResourceID'  OutDataTypeStr=Bus: PRESCAN_VISULIGHTACTUATOR_DATA  NonVirtualBus=on
  Bus Creator1 : BusCreator  Inputs=3  OutDataTypeStr=Bus: PRESCAN_RGB_DATA  NonVirtualBus=on
  Bus Creator2 : BusCreator  Inputs=3  OutDataTypeStr=Bus: PRESCAN_RPY_DATA  NonVirtualBus=on
  Bus Creator3 : BusCreator  Inputs=3  OutDataTypeStr=Bus: PRESCAN_XYZ_DATA  NonVirtualBus=on
  Data Type Conversion : DataTypeConversion  OutDataTypeStr=int32  RndMeth=Nearest
  Degrees to Radians : simulink_extras/Transformations/Degrees to Radians
  Demux : Demux  Outputs=3
  Demux1 : Demux  Outputs=3
  Demux2 : Demux  Outputs=3
  Lights : Outport
  wires:
  TextureResourceID [-]/1 -> Data Type Conversion/1  "TextureResourceID"
  MSCD [Cd]/1 -> Bus Creator/1  "Intensity"
  Bus Creator/1 -> Lights/1
  Demux/1 -> Bus Creator1/1  "R"
  Demux/2 -> Bus Creator1/2  "G"
  Demux/3 -> Bus Creator1/3  "B"
  Color [-]/1 -> Demux/1  "Color"
  Bus Creator1/1 -> Bus Creator/4  "Color"
  Demux1/1 -> Bus Creator2/1  "Roll"
  Demux1/2 -> Bus Creator2/2  "Pitch"
  Demux1/3 -> Bus Creator2/3  "Yaw"
  Orientation (RPY) [deg]/1 -> Degrees to Radians/1  "Orientation"
  Bus Creator2/1 -> Bus Creator/3  "Orientation"
  Demux2/1 -> Bus Creator3/1  "X"
  Demux2/2 -> Bus Creator3/2  "Y"
  Demux2/3 -> Bus Creator3/3  "Z"
  Position (xyz) [m]/1 -> Demux2/1  "Position"
  Bus Creator3/1 -> Bus Creator/2  "Position"
  Data Type Conversion/1 -> Bus Creator/5  "TextureResourceID"
  Degrees to Radians/1 -> Demux1/1

== system W01_Base_Map_cs/TrafficLightRoadSideNL_3/Green_Mux ==
  MSCD [Cd] : Inport
  Position (xyz) [m] : Inport  Port=2
  Orientation (RPY) [deg] : Inport  Port=3
  Color [-] : Inport  Port=4
  TextureResourceID [-] : Inport  Port=5
  Bus Creator : BusCreator  Inputs='Intensity','Position','Orientation','Color','TextureResourceID'  OutDataTypeStr=Bus: PRESCAN_VISULIGHTACTUATOR_DATA  NonVirtualBus=on
  Bus Creator1 : BusCreator  Inputs=3  OutDataTypeStr=Bus: PRESCAN_RGB_DATA  NonVirtualBus=on
  Bus Creator2 : BusCreator  Inputs=3  OutDataTypeStr=Bus: PRESCAN_RPY_DATA  NonVirtualBus=on
  Bus Creator3 : BusCreator  Inputs=3  OutDataTypeStr=Bus: PRESCAN_XYZ_DATA  NonVirtualBus=on
  Data Type Conversion : DataTypeConversion  OutDataTypeStr=int32  RndMeth=Nearest
  Degrees to Radians : simulink_extras/Transformations/Degrees to Radians
  Demux : Demux  Outputs=3
  Demux1 : Demux  Outputs=3
  Demux2 : Demux  Outputs=3
  Lights : Outport
  wires:
  TextureResourceID [-]/1 -> Data Type Conversion/1  "TextureResourceID"
  MSCD [Cd]/1 -> Bus Creator/1  "Intensity"
  Bus Creator/1 -> Lights/1
  Demux/1 -> Bus Creator1/1  "R"
  Demux/2 -> Bus Creator1/2  "G"
  Demux/3 -> Bus Creator1/3  "B"
  Color [-]/1 -> Demux/1  "Color"
  Bus Creator1/1 -> Bus Creator/4  "Color"
  Demux1/1 -> Bus Creator2/1  "Roll"
  Demux1/2 -> Bus Creator2/2  "Pitch"
  Demux1/3 -> Bus Creator2/3  "Yaw"
  Orientation (RPY) [deg]/1 -> Degrees to Radians/1  "Orientation"
  Bus Creator2/1 -> Bus Creator/3  "Orientation"
  Demux2/1 -> Bus Creator3/1  "X"
  Demux2/2 -> Bus Creator3/2  "Y"
  Demux2/3 -> Bus Creator3/3  "Z"
  Position (xyz) [m]/1 -> Demux2/1  "Position"
  Bus Creator3/1 -> Bus Creator/2  "Position"
  Data Type Conversion/1 -> Bus Creator/5  "TextureResourceID"
  Degrees to Radians/1 -> Demux1/1

== system W01_Base_Map_cs/TrafficLightRoadSideNL_3/Orange_Mux ==
  MSCD [Cd] : Inport
  Position (xyz) [m] : Inport  Port=2
  Orientation (RPY) [deg] : Inport  Port=3
  Color [-] : Inport  Port=4
  TextureResourceID [-] : Inport  Port=5
  Bus Creator : BusCreator  Inputs='Intensity','Position','Orientation','Color','TextureResourceID'  OutDataTypeStr=Bus: PRESCAN_VISULIGHTACTUATOR_DATA  NonVirtualBus=on
  Bus Creator1 : BusCreator  Inputs=3  OutDataTypeStr=Bus: PRESCAN_RGB_DATA  NonVirtualBus=on
  Bus Creator2 : BusCreator  Inputs=3  OutDataTypeStr=Bus: PRESCAN_RPY_DATA  NonVirtualBus=on
  Bus Creator3 : BusCreator  Inputs=3  OutDataTypeStr=Bus: PRESCAN_XYZ_DATA  NonVirtualBus=on
  Data Type Conversion : DataTypeConversion  OutDataTypeStr=int32  RndMeth=Nearest
  Degrees to Radians : simulink_extras/Transformations/Degrees to Radians
  Demux : Demux  Outputs=3
  Demux1 : Demux  Outputs=3
  Demux2 : Demux  Outputs=3
  Lights : Outport
  wires:
  TextureResourceID [-]/1 -> Data Type Conversion/1  "TextureResourceID"
  MSCD [Cd]/1 -> Bus Creator/1  "Intensity"
  Bus Creator/1 -> Lights/1
  Demux/1 -> Bus Creator1/1  "R"
  Demux/2 -> Bus Creator1/2  "G"
  Demux/3 -> Bus Creator1/3  "B"
  Color [-]/1 -> Demux/1  "Color"
  Bus Creator1/1 -> Bus Creator/4  "Color"
  Demux1/1 -> Bus Creator2/1  "Roll"
  Demux1/2 -> Bus Creator2/2  "Pitch"
  Demux1/3 -> Bus Creator2/3  "Yaw"
  Orientation (RPY) [deg]/1 -> Degrees to Radians/1  "Orientation"
  Bus Creator2/1 -> Bus Creator/3  "Orientation"
  Demux2/1 -> Bus Creator3/1  "X"
  Demux2/2 -> Bus Creator3/2  "Y"
  Demux2/3 -> Bus Creator3/3  "Z"
  Position (xyz) [m]/1 -> Demux2/1  "Position"
  Bus Creator3/1 -> Bus Creator/2  "Position"
  Data Type Conversion/1 -> Bus Creator/5  "TextureResourceID"
  Degrees to Radians/1 -> Demux1/1

== system W01_Base_Map_cs/TrafficLightRoadSideNL_3/Red_Mux ==
  MSCD [Cd] : Inport
  Position (xyz) [m] : Inport  Port=2
  Orientation (RPY) [deg] : Inport  Port=3
  Color [-] : Inport  Port=4
  TextureResourceID [-] : Inport  Port=5
  Bus Creator : BusCreator  Inputs='Intensity','Position','Orientation','Color','TextureResourceID'  OutDataTypeStr=Bus: PRESCAN_VISULIGHTACTUATOR_DATA  NonVirtualBus=on
  Bus Creator1 : BusCreator  Inputs=3  OutDataTypeStr=Bus: PRESCAN_RGB_DATA  NonVirtualBus=on
  Bus Creator2 : BusCreator  Inputs=3  OutDataTypeStr=Bus: PRESCAN_RPY_DATA  NonVirtualBus=on
  Bus Creator3 : BusCreator  Inputs=3  OutDataTypeStr=Bus: PRESCAN_XYZ_DATA  NonVirtualBus=on
  Data Type Conversion : DataTypeConversion  OutDataTypeStr=int32  RndMeth=Nearest
  Degrees to Radians : simulink_extras/Transformations/Degrees to Radians
  Demux : Demux  Outputs=3
  Demux1 : Demux  Outputs=3
  Demux2 : Demux  Outputs=3
  Lights : Outport
  wires:
  TextureResourceID [-]/1 -> Data Type Conversion/1  "TextureResourceID"
  MSCD [Cd]/1 -> Bus Creator/1  "Intensity"
  Bus Creator/1 -> Lights/1
  Demux/1 -> Bus Creator1/1  "R"
  Demux/2 -> Bus Creator1/2  "G"
  Demux/3 -> Bus Creator1/3  "B"
  Color [-]/1 -> Demux/1  "Color"
  Bus Creator1/1 -> Bus Creator/4  "Color"
  Demux1/1 -> Bus Creator2/1  "Roll"
  Demux1/2 -> Bus Creator2/2  "Pitch"
  Demux1/3 -> Bus Creator2/3  "Yaw"
  Orientation (RPY) [deg]/1 -> Degrees to Radians/1  "Orientation"
  Bus Creator2/1 -> Bus Creator/3  "Orientation"
  Demux2/1 -> Bus Creator3/1  "X"
  Demux2/2 -> Bus Creator3/2  "Y"
  Demux2/3 -> Bus Creator3/3  "Z"
  Position (xyz) [m]/1 -> Demux2/1  "Position"
  Bus Creator3/1 -> Bus Creator/2  "Position"
  Data Type Conversion/1 -> Bus Creator/5  "TextureResourceID"
  Degrees to Radians/1 -> Demux1/1

== system W01_Base_Map_cs/TrafficLightRoadSideNL_4/Green_Mux ==
  MSCD [Cd] : Inport
  Position (xyz) [m] : Inport  Port=2
  Orientation (RPY) [deg] : Inport  Port=3
  Color [-] : Inport  Port=4
  TextureResourceID [-] : Inport  Port=5
  Bus Creator : BusCreator  Inputs='Intensity','Position','Orientation','Color','TextureResourceID'  OutDataTypeStr=Bus: PRESCAN_VISULIGHTACTUATOR_DATA  NonVirtualBus=on
  Bus Creator1 : BusCreator  Inputs=3  OutDataTypeStr=Bus: PRESCAN_RGB_DATA  NonVirtualBus=on
  Bus Creator2 : BusCreator  Inputs=3  OutDataTypeStr=Bus: PRESCAN_RPY_DATA  NonVirtualBus=on
  Bus Creator3 : BusCreator  Inputs=3  OutDataTypeStr=Bus: PRESCAN_XYZ_DATA  NonVirtualBus=on
  Data Type Conversion : DataTypeConversion  OutDataTypeStr=int32  RndMeth=Nearest
  Degrees to Radians : simulink_extras/Transformations/Degrees to Radians
  Demux : Demux  Outputs=3
  Demux1 : Demux  Outputs=3
  Demux2 : Demux  Outputs=3
  Lights : Outport
  wires:
  TextureResourceID [-]/1 -> Data Type Conversion/1  "TextureResourceID"
  MSCD [Cd]/1 -> Bus Creator/1  "Intensity"
  Bus Creator/1 -> Lights/1
  Demux/1 -> Bus Creator1/1  "R"
  Demux/2 -> Bus Creator1/2  "G"
  Demux/3 -> Bus Creator1/3  "B"
  Color [-]/1 -> Demux/1  "Color"
  Bus Creator1/1 -> Bus Creator/4  "Color"
  Demux1/1 -> Bus Creator2/1  "Roll"
  Demux1/2 -> Bus Creator2/2  "Pitch"
  Demux1/3 -> Bus Creator2/3  "Yaw"
  Orientation (RPY) [deg]/1 -> Degrees to Radians/1  "Orientation"
  Bus Creator2/1 -> Bus Creator/3  "Orientation"
  Demux2/1 -> Bus Creator3/1  "X"
  Demux2/2 -> Bus Creator3/2  "Y"
  Demux2/3 -> Bus Creator3/3  "Z"
  Position (xyz) [m]/1 -> Demux2/1  "Position"
  Bus Creator3/1 -> Bus Creator/2  "Position"
  Data Type Conversion/1 -> Bus Creator/5  "TextureResourceID"
  Degrees to Radians/1 -> Demux1/1

== system W01_Base_Map_cs/TrafficLightRoadSideNL_4/Orange_Mux ==
  MSCD [Cd] : Inport
  Position (xyz) [m] : Inport  Port=2
  Orientation (RPY) [deg] : Inport  Port=3
  Color [-] : Inport  Port=4
  TextureResourceID [-] : Inport  Port=5
  Bus Creator : BusCreator  Inputs='Intensity','Position','Orientation','Color','TextureResourceID'  OutDataTypeStr=Bus: PRESCAN_VISULIGHTACTUATOR_DATA  NonVirtualBus=on
  Bus Creator1 : BusCreator  Inputs=3  OutDataTypeStr=Bus: PRESCAN_RGB_DATA  NonVirtualBus=on
  Bus Creator2 : BusCreator  Inputs=3  OutDataTypeStr=Bus: PRESCAN_RPY_DATA  NonVirtualBus=on
  Bus Creator3 : BusCreator  Inputs=3  OutDataTypeStr=Bus: PRESCAN_XYZ_DATA  NonVirtualBus=on
  Data Type Conversion : DataTypeConversion  OutDataTypeStr=int32  RndMeth=Nearest
  Degrees to Radians : simulink_extras/Transformations/Degrees to Radians
  Demux : Demux  Outputs=3
  Demux1 : Demux  Outputs=3
  Demux2 : Demux  Outputs=3
  Lights : Outport
  wires:
  TextureResourceID [-]/1 -> Data Type Conversion/1  "TextureResourceID"
  MSCD [Cd]/1 -> Bus Creator/1  "Intensity"
  Bus Creator/1 -> Lights/1
  Demux/1 -> Bus Creator1/1  "R"
  Demux/2 -> Bus Creator1/2  "G"
  Demux/3 -> Bus Creator1/3  "B"
  Color [-]/1 -> Demux/1  "Color"
  Bus Creator1/1 -> Bus Creator/4  "Color"
  Demux1/1 -> Bus Creator2/1  "Roll"
  Demux1/2 -> Bus Creator2/2  "Pitch"
  Demux1/3 -> Bus Creator2/3  "Yaw"
  Orientation (RPY) [deg]/1 -> Degrees to Radians/1  "Orientation"
  Bus Creator2/1 -> Bus Creator/3  "Orientation"
  Demux2/1 -> Bus Creator3/1  "X"
  Demux2/2 -> Bus Creator3/2  "Y"
  Demux2/3 -> Bus Creator3/3  "Z"
  Position (xyz) [m]/1 -> Demux2/1  "Position"
  Bus Creator3/1 -> Bus Creator/2  "Position"
  Data Type Conversion/1 -> Bus Creator/5  "TextureResourceID"
  Degrees to Radians/1 -> Demux1/1

== system W01_Base_Map_cs/TrafficLightRoadSideNL_4/Red_Mux ==
  MSCD [Cd] : Inport
  Position (xyz) [m] : Inport  Port=2
  Orientation (RPY) [deg] : Inport  Port=3
  Color [-] : Inport  Port=4
  TextureResourceID [-] : Inport  Port=5
  Bus Creator : BusCreator  Inputs='Intensity','Position','Orientation','Color','TextureResourceID'  OutDataTypeStr=Bus: PRESCAN_VISULIGHTACTUATOR_DATA  NonVirtualBus=on
  Bus Creator1 : BusCreator  Inputs=3  OutDataTypeStr=Bus: PRESCAN_RGB_DATA  NonVirtualBus=on
  Bus Creator2 : BusCreator  Inputs=3  OutDataTypeStr=Bus: PRESCAN_RPY_DATA  NonVirtualBus=on
  Bus Creator3 : BusCreator  Inputs=3  OutDataTypeStr=Bus: PRESCAN_XYZ_DATA  NonVirtualBus=on
  Data Type Conversion : DataTypeConversion  OutDataTypeStr=int32  RndMeth=Nearest
  Degrees to Radians : simulink_extras/Transformations/Degrees to Radians
  Demux : Demux  Outputs=3
  Demux1 : Demux  Outputs=3
  Demux2 : Demux  Outputs=3
  Lights : Outport
  wires:
  TextureResourceID [-]/1 -> Data Type Conversion/1  "TextureResourceID"
  MSCD [Cd]/1 -> Bus Creator/1  "Intensity"
  Bus Creator/1 -> Lights/1
  Demux/1 -> Bus Creator1/1  "R"
  Demux/2 -> Bus Creator1/2  "G"
  Demux/3 -> Bus Creator1/3  "B"
  Color [-]/1 -> Demux/1  "Color"
  Bus Creator1/1 -> Bus Creator/4  "Color"
  Demux1/1 -> Bus Creator2/1  "Roll"
  Demux1/2 -> Bus Creator2/2  "Pitch"
  Demux1/3 -> Bus Creator2/3  "Yaw"
  Orientation (RPY) [deg]/1 -> Degrees to Radians/1  "Orientation"
  Bus Creator2/1 -> Bus Creator/3  "Orientation"
  Demux2/1 -> Bus Creator3/1  "X"
  Demux2/2 -> Bus Creator3/2  "Y"
  Demux2/3 -> Bus Creator3/3  "Z"
  Position (xyz) [m]/1 -> Demux2/1  "Position"
  Bus Creator3/1 -> Bus Creator/2  "Position"
  Data Type Conversion/1 -> Bus Creator/5  "TextureResourceID"
  Degrees to Radians/1 -> Demux1/1

== system W01_Base_Map_cs/TrafficLightRoadSideNL_5/Green_Mux ==
  MSCD [Cd] : Inport
  Position (xyz) [m] : Inport  Port=2
  Orientation (RPY) [deg] : Inport  Port=3
  Color [-] : Inport  Port=4
  TextureResourceID [-] : Inport  Port=5
  Bus Creator : BusCreator  Inputs='Intensity','Position','Orientation','Color','TextureResourceID'  OutDataTypeStr=Bus: PRESCAN_VISULIGHTACTUATOR_DATA  NonVirtualBus=on
  Bus Creator1 : BusCreator  Inputs=3  OutDataTypeStr=Bus: PRESCAN_RGB_DATA  NonVirtualBus=on
  Bus Creator2 : BusCreator  Inputs=3  OutDataTypeStr=Bus: PRESCAN_RPY_DATA  NonVirtualBus=on
  Bus Creator3 : BusCreator  Inputs=3  OutDataTypeStr=Bus: PRESCAN_XYZ_DATA  NonVirtualBus=on
  Data Type Conversion : DataTypeConversion  OutDataTypeStr=int32  RndMeth=Nearest
  Degrees to Radians : simulink_extras/Transformations/Degrees to Radians
  Demux : Demux  Outputs=3
  Demux1 : Demux  Outputs=3
  Demux2 : Demux  Outputs=3
  Lights : Outport
  wires:
  TextureResourceID [-]/1 -> Data Type Conversion/1  "TextureResourceID"
  MSCD [Cd]/1 -> Bus Creator/1  "Intensity"
  Bus Creator/1 -> Lights/1
  Demux/1 -> Bus Creator1/1  "R"
  Demux/2 -> Bus Creator1/2  "G"
  Demux/3 -> Bus Creator1/3  "B"
  Color [-]/1 -> Demux/1  "Color"
  Bus Creator1/1 -> Bus Creator/4  "Color"
  Demux1/1 -> Bus Creator2/1  "Roll"
  Demux1/2 -> Bus Creator2/2  "Pitch"
  Demux1/3 -> Bus Creator2/3  "Yaw"
  Orientation (RPY) [deg]/1 -> Degrees to Radians/1  "Orientation"
  Bus Creator2/1 -> Bus Creator/3  "Orientation"
  Demux2/1 -> Bus Creator3/1  "X"
  Demux2/2 -> Bus Creator3/2  "Y"
  Demux2/3 -> Bus Creator3/3  "Z"
  Position (xyz) [m]/1 -> Demux2/1  "Position"
  Bus Creator3/1 -> Bus Creator/2  "Position"
  Data Type Conversion/1 -> Bus Creator/5  "TextureResourceID"
  Degrees to Radians/1 -> Demux1/1

== system W01_Base_Map_cs/TrafficLightRoadSideNL_5/Orange_Mux ==
  MSCD [Cd] : Inport
  Position (xyz) [m] : Inport  Port=2
  Orientation (RPY) [deg] : Inport  Port=3
  Color [-] : Inport  Port=4
  TextureResourceID [-] : Inport  Port=5
  Bus Creator : BusCreator  Inputs='Intensity','Position','Orientation','Color','TextureResourceID'  OutDataTypeStr=Bus: PRESCAN_VISULIGHTACTUATOR_DATA  NonVirtualBus=on
  Bus Creator1 : BusCreator  Inputs=3  OutDataTypeStr=Bus: PRESCAN_RGB_DATA  NonVirtualBus=on
  Bus Creator2 : BusCreator  Inputs=3  OutDataTypeStr=Bus: PRESCAN_RPY_DATA  NonVirtualBus=on
  Bus Creator3 : BusCreator  Inputs=3  OutDataTypeStr=Bus: PRESCAN_XYZ_DATA  NonVirtualBus=on
  Data Type Conversion : DataTypeConversion  OutDataTypeStr=int32  RndMeth=Nearest
  Degrees to Radians : simulink_extras/Transformations/Degrees to Radians
  Demux : Demux  Outputs=3
  Demux1 : Demux  Outputs=3
  Demux2 : Demux  Outputs=3
  Lights : Outport
  wires:
  TextureResourceID [-]/1 -> Data Type Conversion/1  "TextureResourceID"
  MSCD [Cd]/1 -> Bus Creator/1  "Intensity"
  Bus Creator/1 -> Lights/1
  Demux/1 -> Bus Creator1/1  "R"
  Demux/2 -> Bus Creator1/2  "G"
  Demux/3 -> Bus Creator1/3  "B"
  Color [-]/1 -> Demux/1  "Color"
  Bus Creator1/1 -> Bus Creator/4  "Color"
  Demux1/1 -> Bus Creator2/1  "Roll"
  Demux1/2 -> Bus Creator2/2  "Pitch"
  Demux1/3 -> Bus Creator2/3  "Yaw"
  Orientation (RPY) [deg]/1 -> Degrees to Radians/1  "Orientation"
  Bus Creator2/1 -> Bus Creator/3  "Orientation"
  Demux2/1 -> Bus Creator3/1  "X"
  Demux2/2 -> Bus Creator3/2  "Y"
  Demux2/3 -> Bus Creator3/3  "Z"
  Position (xyz) [m]/1 -> Demux2/1  "Position"
  Bus Creator3/1 -> Bus Creator/2  "Position"
  Data Type Conversion/1 -> Bus Creator/5  "TextureResourceID"
  Degrees to Radians/1 -> Demux1/1

== system W01_Base_Map_cs/TrafficLightRoadSideNL_5/Red_Mux ==
  MSCD [Cd] : Inport
  Position (xyz) [m] : Inport  Port=2
  Orientation (RPY) [deg] : Inport  Port=3
  Color [-] : Inport  Port=4
  TextureResourceID [-] : Inport  Port=5
  Bus Creator : BusCreator  Inputs='Intensity','Position','Orientation','Color','TextureResourceID'  OutDataTypeStr=Bus: PRESCAN_VISULIGHTACTUATOR_DATA  NonVirtualBus=on
  Bus Creator1 : BusCreator  Inputs=3  OutDataTypeStr=Bus: PRESCAN_RGB_DATA  NonVirtualBus=on
  Bus Creator2 : BusCreator  Inputs=3  OutDataTypeStr=Bus: PRESCAN_RPY_DATA  NonVirtualBus=on
  Bus Creator3 : BusCreator  Inputs=3  OutDataTypeStr=Bus: PRESCAN_XYZ_DATA  NonVirtualBus=on
  Data Type Conversion : DataTypeConversion  OutDataTypeStr=int32  RndMeth=Nearest
  Degrees to Radians : simulink_extras/Transformations/Degrees to Radians
  Demux : Demux  Outputs=3
  Demux1 : Demux  Outputs=3
  Demux2 : Demux  Outputs=3
  Lights : Outport
  wires:
  TextureResourceID [-]/1 -> Data Type Conversion/1  "TextureResourceID"
  MSCD [Cd]/1 -> Bus Creator/1  "Intensity"
  Bus Creator/1 -> Lights/1
  Demux/1 -> Bus Creator1/1  "R"
  Demux/2 -> Bus Creator1/2  "G"
  Demux/3 -> Bus Creator1/3  "B"
  Color [-]/1 -> Demux/1  "Color"
  Bus Creator1/1 -> Bus Creator/4  "Color"
  Demux1/1 -> Bus Creator2/1  "Roll"
  Demux1/2 -> Bus Creator2/2  "Pitch"
  Demux1/3 -> Bus Creator2/3  "Yaw"
  Orientation (RPY) [deg]/1 -> Degrees to Radians/1  "Orientation"
  Bus Creator2/1 -> Bus Creator/3  "Orientation"
  Demux2/1 -> Bus Creator3/1  "X"
  Demux2/2 -> Bus Creator3/2  "Y"
  Demux2/3 -> Bus Creator3/3  "Z"
  Position (xyz) [m]/1 -> Demux2/1  "Position"
  Bus Creator3/1 -> Bus Creator/2  "Position"
  Data Type Conversion/1 -> Bus Creator/5  "TextureResourceID"
  Degrees to Radians/1 -> Demux1/1

== system W01_Base_Map_cs/TrafficLightRoadSideNL_6/Green_Mux ==
  MSCD [Cd] : Inport
  Position (xyz) [m] : Inport  Port=2
  Orientation (RPY) [deg] : Inport  Port=3
  Color [-] : Inport  Port=4
  TextureResourceID [-] : Inport  Port=5
  Bus Creator : BusCreator  Inputs='Intensity','Position','Orientation','Color','TextureResourceID'  OutDataTypeStr=Bus: PRESCAN_VISULIGHTACTUATOR_DATA  NonVirtualBus=on
  Bus Creator1 : BusCreator  Inputs=3  OutDataTypeStr=Bus: PRESCAN_RGB_DATA  NonVirtualBus=on
  Bus Creator2 : BusCreator  Inputs=3  OutDataTypeStr=Bus: PRESCAN_RPY_DATA  NonVirtualBus=on
  Bus Creator3 : BusCreator  Inputs=3  OutDataTypeStr=Bus: PRESCAN_XYZ_DATA  NonVirtualBus=on
  Data Type Conversion : DataTypeConversion  OutDataTypeStr=int32  RndMeth=Nearest
  Degrees to Radians : simulink_extras/Transformations/Degrees to Radians
  Demux : Demux  Outputs=3
  Demux1 : Demux  Outputs=3
  Demux2 : Demux  Outputs=3
  Lights : Outport
  wires:
  TextureResourceID [-]/1 -> Data Type Conversion/1  "TextureResourceID"
  MSCD [Cd]/1 -> Bus Creator/1  "Intensity"
  Bus Creator/1 -> Lights/1
  Demux/1 -> Bus Creator1/1  "R"
  Demux/2 -> Bus Creator1/2  "G"
  Demux/3 -> Bus Creator1/3  "B"
  Color [-]/1 -> Demux/1  "Color"
  Bus Creator1/1 -> Bus Creator/4  "Color"
  Demux1/1 -> Bus Creator2/1  "Roll"
  Demux1/2 -> Bus Creator2/2  "Pitch"
  Demux1/3 -> Bus Creator2/3  "Yaw"
  Orientation (RPY) [deg]/1 -> Degrees to Radians/1  "Orientation"
  Bus Creator2/1 -> Bus Creator/3  "Orientation"
  Demux2/1 -> Bus Creator3/1  "X"
  Demux2/2 -> Bus Creator3/2  "Y"
  Demux2/3 -> Bus Creator3/3  "Z"
  Position (xyz) [m]/1 -> Demux2/1  "Position"
  Bus Creator3/1 -> Bus Creator/2  "Position"
  Data Type Conversion/1 -> Bus Creator/5  "TextureResourceID"
  Degrees to Radians/1 -> Demux1/1
